simulink model "step_pid"  (R2024b)
settings: Solver=VariableStepAuto  StartTime=0.0  StopTime=10.0  RelTol=1e-3
undefined symbols (not defined in the file or in its folder): den_pid, denP, num_pid, numP
settings Model: Creator=andre  LastModifiedBy=andre

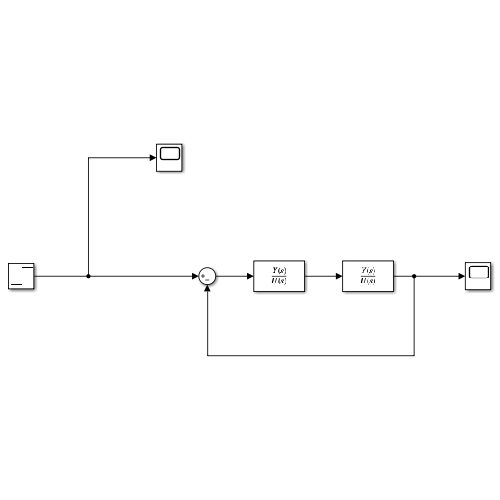
[thumbnail: Simulink's stored preview of the top-level diagram]
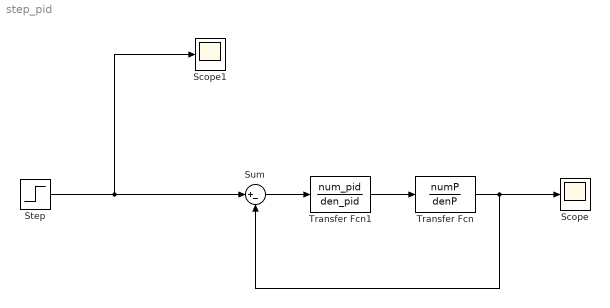
== system step_pid ==
  Scope : Scope
  Scope1 : Scope
  Step : Step  SampleTime=0
  Sum : Sum  Inputs=|+-
  Transfer Fcn : TransferFcn  Numerator=numP  Denominator=denP
  Transfer Fcn1 : TransferFcn  Numerator=num_pid  Denominator=den_pid
  wires:
  Step/1 -> Scope1/1, Sum/1
  Transfer Fcn/1 -> Scope/1, Sum/2
  Sum/1 -> Transfer Fcn1/1
  Transfer Fcn1/1 -> Transfer Fcn/1
